simulink model "Project_Papi_Rubber_Game_SSObs_Sim"  (R2019a)
settings: Solver=FixedStepAuto  StartTime=0.0  StopTime=50  FixedStep=0.01  RelTol=1e-3
undefined symbols (not defined in the file): A, B, C, ene, init_cond, K_int, K_ss, L_obs, m, slop
libraries: simulink x2
settings Model: Creator=asjos  LastModifiedBy=asjos

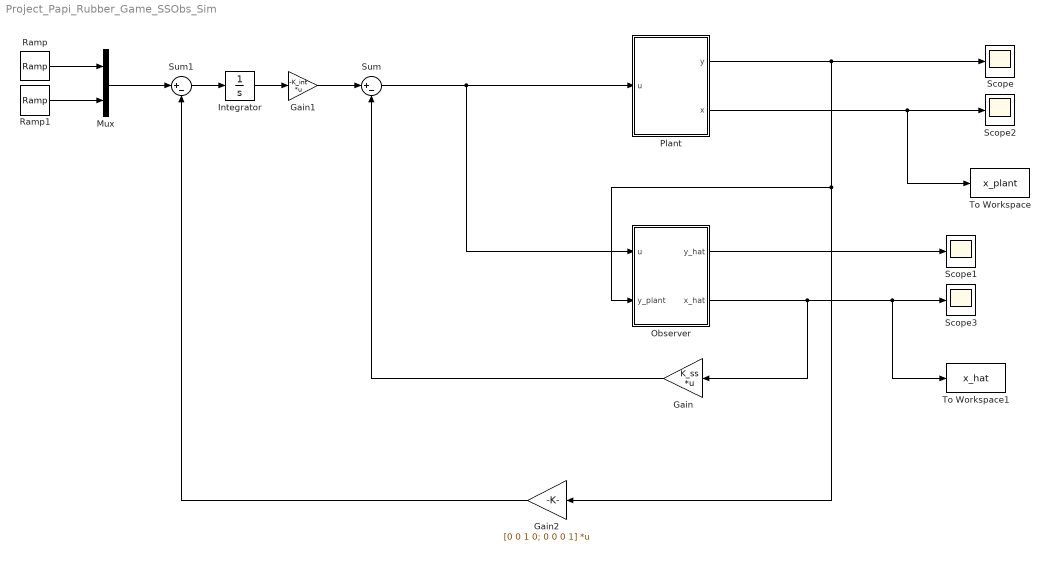
== system Project_Papi_Rubber_Game_SSObs_Sim ==
  Gain : Gain  Gain=K_ss  Multiplication=Matrix(K*u)
  Gain1 : Gain  Gain=-K_int  Multiplication=Matrix(K*u)
  Gain2 : Gain  Gain=[0 0 1 0; 0 0 0 1]  Multiplication=Matrix(K*u)
  Integrator : Integrator  InitialCondition=zeros(2,1)
  Mux : Mux  Inputs=2
  Observer : Subsystem
  Plant : Subsystem
  Ramp : simulink/Sources/Ramp  slope=slop(1,m)  start=0  InitialOutput=ene(1,1)
  Ramp1 : simulink/Sources/Ramp  slope=slop(1,m)  start=0  InitialOutput=ene(1,2)
  Scope{,1..3} (4 alike) : Scope
  Sum : Sum  Inputs=|+-
  Sum1 : Sum  Inputs=|+-
  To Workspace : ToWorkspace  VariableName=x_plant  SaveFormat=Timeseries  SampleTime=-1
  To Workspace1 : ToWorkspace  VariableName=x_hat  SaveFormat=Timeseries  SampleTime=-1
  wires:
  Plant/1(y) -> Gain2/1, Observer/2(y_plant), Scope/1
  Sum/1 -> Observer/1(u), Plant/1(u)
  Gain/1 -> Sum/2
  Observer/2(x_hat) -> To Workspace1/1, Scope3/1, Gain/1
  Observer/1(y_hat) -> Scope1/1
  Plant/2(x) -> To Workspace/1, Scope2/1
  Ramp/1 -> Mux/1
  Ramp1/1 -> Mux/2
  Mux/1 -> Sum1/1
  Sum1/1 -> Integrator/1
  Gain1/1 -> Sum/1
  Integrator/1 -> Gain1/1
  Gain2/1 -> Sum1/2

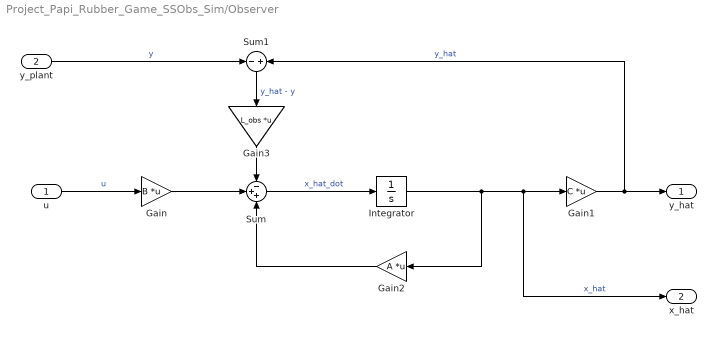
== system Project_Papi_Rubber_Game_SSObs_Sim/Observer ==
  u : Inport
  y_plant : Inport  Port=2
  Gain : Gain  Gain=B  Multiplication=Matrix(K*u)
  Gain1 : Gain  Gain=C  Multiplication=Matrix(K*u)
  Gain2 : Gain  Gain=A  Multiplication=Matrix(K*u)
  Gain3 : Gain  Gain=L_obs  Multiplication=Matrix(K*u)
  Integrator : Integrator  InitialCondition=init_cond
  Sum : Sum  Inputs=-++
  Sum1 : Sum  Inputs=-|+
  y_hat : Outport
  x_hat : Outport  Port=2
  wires:
  Integrator/1 -> x_hat/1, Gain1/1, Gain2/1  "x_hat"
  Sum/1 -> Integrator/1  "x_hat_dot"
  u/1 -> Gain/1  "u"
  Gain1/1 -> Sum1/2, y_hat/1  "y_hat"
  Gain/1 -> Sum/2
  Gain2/1 -> Sum/3
  y_plant/1 -> Sum1/1  "y"
  Sum1/1 -> Gain3/1  "y_hat - y"
  Gain3/1 -> Sum/1

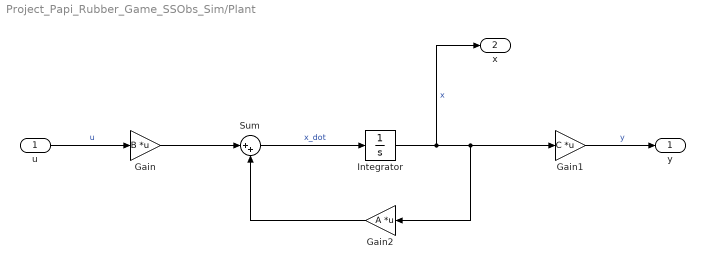
== system Project_Papi_Rubber_Game_SSObs_Sim/Plant ==
  u : Inport
  Gain : Gain  Gain=B  Multiplication=Matrix(K*u)
  Gain1 : Gain  Gain=C  Multiplication=Matrix(K*u)
  Gain2 : Gain  Gain=A  Multiplication=Matrix(K*u)
  Integrator : Integrator  InitialCondition=init_cond
  Sum : Sum  Inputs=|++
  y : Outport
  x : Outport  Port=2
  wires:
  Integrator/1 -> x/1, Gain1/1, Gain2/1  "x"
  Gain2/1 -> Sum/2
  Gain/1 -> Sum/1
  Sum/1 -> Integrator/1  "x_dot"
  u/1 -> Gain/1  "u"
  Gain1/1 -> y/1  "y"
